simulink model "Observador_clasico_discreto_plantilla"  (R2016a)
settings: Solver=VariableStepAuto  StartTime=0.0  StopTime=10  RelTol=1e-3
values from neighbouring files (symbols this model uses):
  ki = k(1:1,3:3)    [Regulador_seguidor_observador_codigo.m]
  tm = 0.1    [Regulador_seguidor_observador_codigo.m]
undefined symbols (not defined in the file or in its folder): A_dis, B_dis, C_dis, denu_dis, deny_dis, numu_dis, numy_dis
settings Model: Creator=Daniel  LastModifiedBy=Daniel

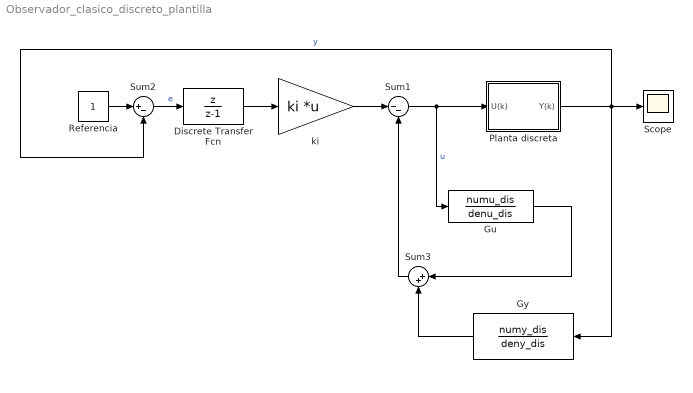
== system Observador_clasico_discreto_plantilla ==
  Discrete Transfer Fcn : DiscreteTransferFcn  Numerator=[1 0]  Denominator=[1 -1]  SampleTime=tm
  Gu : TransferFcn  Numerator=numu_dis  Denominator=denu_dis
  Gy : TransferFcn  Numerator=numy_dis  Denominator=deny_dis
  Planta discreta : Subsystem
  Referencia : Constant
  Scope : Scope
  Sum1 : Sum  Inputs=|--
  Sum2 : Sum  Inputs=|+-
  Sum3 : Sum  Inputs=|++
  ki : Gain  Gain=ki  Multiplication=Matrix(K*u) (u vector)
  wires:
  Planta discreta/1(Y(k)) -> Scope/1, Gy/1, Sum2/2  "y"
  Sum1/1 -> Planta discreta/1(U(k)), Gu/1  "u"
  Discrete Transfer Fcn/1 -> ki/1
  Sum2/1 -> Discrete Transfer Fcn/1  "e"
  Referencia/1 -> Sum2/1
  ki/1 -> Sum1/1
  Gu/1 -> Sum3/1
  Gy/1 -> Sum3/2
  Sum3/1 -> Sum1/2

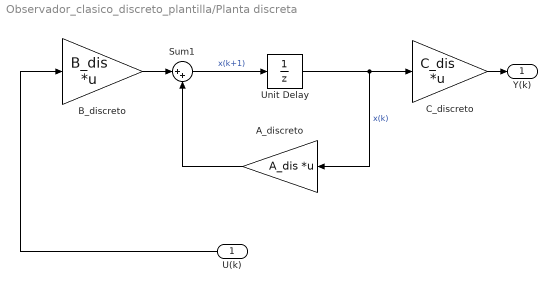
== system Observador_clasico_discreto_plantilla/Planta discreta ==
  U(k) : Inport
  A_discreto : Gain  Gain=A_dis  Multiplication=Matrix(K*u) (u vector)
  B_discreto : Gain  Gain=B_dis  Multiplication=Matrix(K*u) (u vector)
  C_discreto : Gain  Gain=C_dis  Multiplication=Matrix(K*u) (u vector)
  Sum1 : Sum  Inputs=|++
  Unit Delay : UnitDelay  InitialCondition=[1;1]  SampleTime=tm
  Y(k) : Outport
  wires:
  Unit Delay/1 -> A_discreto/1, C_discreto/1  "x(k)"
  A_discreto/1 -> Sum1/2
  Sum1/1 -> Unit Delay/1  "x(k+1)"
  C_discreto/1 -> Y(k)/1
  U(k)/1 -> B_discreto/1
  B_discreto/1 -> Sum1/1
